simulink model "BoatSim"  (R2018a)
settings: Solver=ode45  StartTime=0.0  StopTime=50  RelTol=1e-3  EnableMultiTasking=on
values from neighbouring files (symbols this model uses):
  Dr = 30000    [BoatSim_config.m]
  Du = 1000    [BoatSim_config.m]
  Dv = 10000    [BoatSim_config.m]
  IoM = ( 1 / 5 ) * Mass * ( ( Length / 2 )^2 + ( Width / 2 )^2 )    (= 4143.75)    [BoatSim_config.m]
  Mass = 1500    [BoatSim_config.m]
  rg = [ 0;0; ]    [BoatSim_config.m]
undefined symbols (not defined in the file or in its folder): OM, sigbuilder_block
libraries: simulink x1
settings Model: Creator=hamada  LastModifiedBy=ryodo
settings DataIOCC: LimitDataPoints=on  SaveFormat=Array
settings OptimizationCC: LifeSpan=inf
settings DebuggingCC: SFUnexpectedBacktrackingDiag=warning  SFNoUnconditionalDefaultTransitionDiag=warning  SFExecutionAtInitializationDiag=none
settings HardwareCC: ProdBitPerPointer=32  ProdBitPerSizeT=32  ProdBitPerPtrDiffT=32  ProdLargestAtomicFloat=None  ProdIntDivRoundTo=Undefined  ProdEndianess=Unspecified  ProdWordSize=32  ProdHWDeviceType=32-bit Generic
settings ModelReferenceCC: PropagateSignalLabelsOutOfModel=off
settings CodeAppCC: StateflowObjectComments=on
settings GRTTargetCC: TargetLangStandard=C89/C90 (ANSI)  GeneratePreprocessorConditionals=Disable all
settings ConfigComp: CovMetricSettings=dw  CovHtmlReporting=on  CovSaveCumulativeToWorkspaceVar=on  CovSaveSingleToWorkspaceVar=on  CovExternalEMLEnable=off

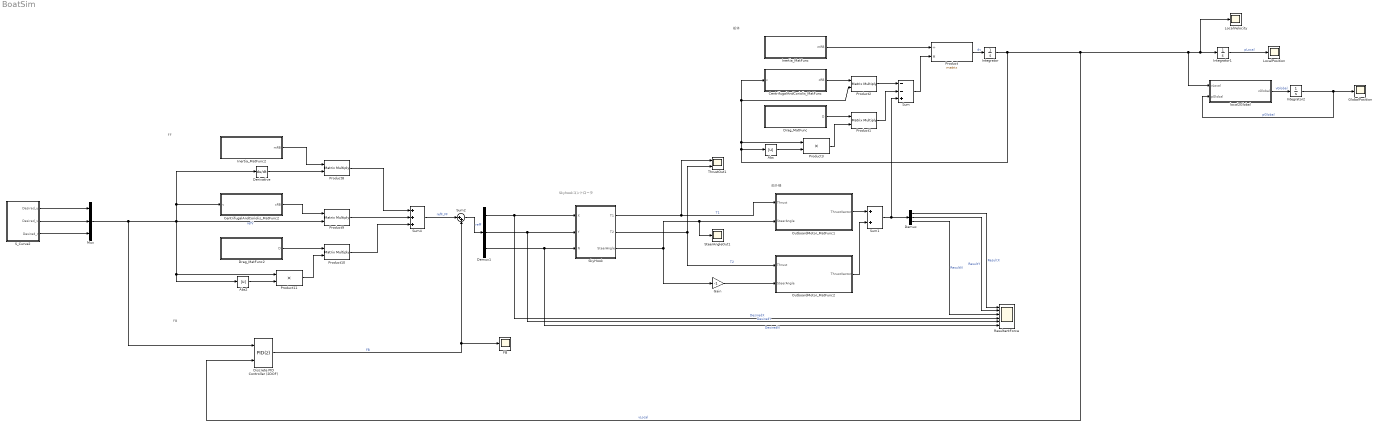
== system BoatSim ==
  note: 船外機
  note: 船体
  note: Skyhookコントローラ
  note: FF
  note: FB
  Abs : Abs
  Abs2 : Abs
  CentrifugalAndCoriolis_MatFunc : MATLAB Function  TreatAsAtomicUnit=on
  CentrifugalAndCoriolis_MatFunc2 : MATLAB Function  TreatAsAtomicUnit=on
  Demux : Demux  Outputs=3
  Demux1 : Demux  Outputs=3
  Derivative : Derivative
  Discrete PID Controller (2DOF) : simulink/Continuous/PID Controller (2DOF)  Controller=PID  TimeDomain=Discrete-time  SampleTime=-1  IntegratorMethod=Forward Euler  FilterMethod=Forward Euler  Form=Parallel  UseFilter=on  ControllerParametersSource=internal  P=1000  I=0  D=0  N=100  b=1  c=1  InitialConditionSource=internal  InitialConditionForIntegrator=0  InitialConditionForFilter=0  ExternalReset=none  ZeroCross=off  LimitOutput=off  UpperSaturationLimit=inf  LowerSaturationLimit=-inf  LinearizeAsGain=off  AntiWindupMode=none  Kb=1  TrackingMode=off  Kt=1  PParamMin=[]  PParamMax=[]  IParamMin=[]  IParamMax=[]  DParamMin=[]  DParamMax=[]  NParamMin=[]  NParamMax=[]  bParamMin=[]  bParamMax=[]  cParamMin=[]  cParamMax=[]  KbParamMin=[]  KbParamMax=[]  KtParamMin=[]  KtParamMax=[]  POutMin=[]  POutMax=[]  IOutMin=[]  IOutMax=[]  DOutMin=[]  DOutMax=[]  NOutMin=[]  NOutMax=[]  bOutMin=[]  bOutMax=[]  cOutMin=[]  cOutMax=[]  KbOutMin=[]  KbOutMax=[]  KtOutMin=[]  KtOutMax=[]  IntegratorOutMin=[]  IntegratorOutMax=[]  FilterOutMin=[]  FilterOutMax=[]  SumOutMin=[]  SumOutMax=[]  Sum1OutMin=[]  Sum1OutMax=[]  Sum2OutMin=[]  Sum2OutMax=[]  Sum3OutMin=[]  Sum3OutMax=[]  SumI1OutMin=[]  SumI1OutMax=[]  SumI2OutMin=[]  SumI2OutMax=[]  SumI3OutMin=[]  SumI3OutMax=[]  SumDOutMin=[]  SumDOutMax=[]  SaturationOutMin=[]  SaturationOutMax=[]  IntegratorContinuousStateAttributes=''  IntegratorStateMustResolveToSignalObject=off  IntegratorRTWStateStorageClass=Auto  FilterContinuousStateAttributes=''  FilterStateMustResolveToSignalObject=off  FilterRTWStateStorageClass=Auto  DifferentiatorICPrevScaledInput=0  DifferentiatorOutMin=[]  DifferentiatorOutMax=[]  FilterDiffOutCoefMin=[]  FilterDiffOutCoefMax=[]  SumDenOutMin=[]  SumDenOutMax=[]  SumNumOutMin=[]  SumNumOutMax=[]  ReciprocalOutMin=[]  ReciprocalOutMax=[]  DivideOutMin=[]  DivideOutMax=[]  TunerSelectOption=Transfer Function Based (PID Tuner App)
  Drag_MatFunc : MATLAB Function  TreatAsAtomicUnit=on  SystemSampleTime=0
      settings: MinAlgLoopOccurrences=on
  Drag_MatFunc2 : MATLAB Function  TreatAsAtomicUnit=on
  FB : Scope
  Gain : Gain  Gain=-1
  GlobalPosition : Scope
  Inertia_MatFunc : MATLAB Function  TreatAsAtomicUnit=on  SystemSampleTime=0
  Inertia_MatFunc2 : MATLAB Function  TreatAsAtomicUnit=on
  Integrator : Integrator
  Integrator1 : Integrator
  Integrator2 : Integrator
  LocalPosition : Scope
  "LocalVelocity " : Scope
  Mux : Mux  Inputs=3
  OutboardMotor_MatFunc1 : MATLAB Function  TreatAsAtomicUnit=on
  OutboardMotor_MatFunc2 : MATLAB Function  TreatAsAtomicUnit=on
  Product : Product  Inputs=/*  Multiplication=Matrix(*)
  Product{1..2,8..10} (5 alike) : Product  Multiplication=Matrix(*)
  Product11 : Product
  Product3 : Product
  ResultantForce : Scope  NumInputPorts=6
  S_Curve2 : Subsystem  Tag=STV Subsys  LoadFcn=sigbuilder_block('load',[244.8 146.274 948.126 560.842 ]);  StartFcn=sigbuilder_block('start');  StopFcn=sigbuilder_block('stop');  ClipboardFcn=sigbuilder_block('clipboard');  mask(Sigbuilder block){tuvar=[0:10]}
      mask help: Simulink:masks:SigbuilderBlock_MD
      mask init:
      | if ~strcmp(get_param(bdroot(gcbh),'SimulationStatus'),'stopped') tuvar = sigbuilder_block('maskInit'); end
      settings: CopyFcn=sigbuilder_block('copy');  DeleteFcn=sigbuilder_block('delete');  ModelCloseFcn=sigbuilder_block('modelClose');  PreSaveFcn=sigbuilder_block('preSave');  PauseFcn=sigbuilder_block('pause');  ContinueFcn=sigbuilder_block('continue');  NameChangeFcn=sigbuilder_block('namechange');  OpenFcn=sigbuilder_block('open',[674 298 550 400 ]);  CloseFcn=sigbuilder_block('close');
      mask Display: plot(0, 0, 100, 100,[2, 2, 32, 32, 2], [68, 8, 8, 68, 68],[32, 2], [38, 38], [32, 19, 2],[53, 60, 44], [32, 17, 17, 2],[16, 16, 31, 31]);txt = getActiveGroup(gcbh);text(2, 100, txt,'verticalAlignment', 'top');
  "SkyHook " : MATLAB Function  TreatAsAtomicUnit=on
  SteerAngleOut1 : Scope
  Sum : Sum  Inputs=--+
  Sum1 : Sum
  Sum2 : Sum  Inputs=|++
  Sum4 : Sum  Inputs=+++
  ThrustOut1 : Scope  NumInputPorts=2
  local2Global : MATLAB Function  TreatAsAtomicUnit=on
  wires:
  Inertia_MatFunc/1(mRB) -> Product/1
  Product/1 -> Integrator/1  "dv"
  Integrator/1 -> Discrete PID Controller (2DOF)/2, local2Global/1(vLocal), "LocalVelocity "/1, Integrator1/1, Abs/1, Product3/1, CentrifugalAndCoriolis_MatFunc/1(v), Product2/2  "vLocal"
  Integrator1/1 -> LocalPosition/1  "pLocal"
  CentrifugalAndCoriolis_MatFunc/1(cRB) -> Product2/1
  Product2/1 -> Sum/1
  Drag_MatFunc/1(D) -> Product1/1
  Sum/1 -> Product/2
  local2Global/1(vGlobal) -> Integrator2/1  "vGlobal"
  Integrator2/1 -> local2Global/2(pGlobal), GlobalPosition/1  "pGlobal"
  Sum1/1 -> Demux/1, Sum/3
  OutboardMotor_MatFunc1/1(ThrustVector) -> Sum1/1
  OutboardMotor_MatFunc2/1(ThrustVector) -> Sum1/2
  Demux/1 -> ResultantForce/1  "ResultX"
  Demux/2 -> ResultantForce/2  "ResultY"
  Demux/3 -> ResultantForce/3  "ResultN"
  Product1/1 -> Sum/2
  Product3/1 -> Product1/2
  Abs/1 -> Product3/2
  S_Curve2/1(Desired_u) -> Mux/1
  S_Curve2/2(Desired_v) -> Mux/2
  S_Curve2/3(Desired_r) -> Mux/3
  Inertia_MatFunc2/1(mRB) -> Product8/1
  Derivative/1 -> Product8/2
  CentrifugalAndCoriolis_MatFunc2/1(cRB) -> Product9/1
  Abs2/1 -> Product11/2
  Mux/1 -> Discrete PID Controller (2DOF)/1, Product11/1, Abs2/1, Derivative/1, CentrifugalAndCoriolis_MatFunc2/1(v), Product9/2  "refV"
  Product11/1 -> Product10/2
  Drag_MatFunc2/1(D) -> Product10/1
  Product8/1 -> Sum4/1
  Product9/1 -> Sum4/2
  Product10/1 -> Sum4/3
  Demux1/1 -> ResultantForce/4, "SkyHook "/1(X)  "DesiredX"
  Demux1/3 -> ResultantForce/6, "SkyHook "/3(N)  "DesiredN"
  Sum4/1 -> Sum2/1  "refF_FF"
  Demux1/2 -> "SkyHook "/2(Y), ResultantForce/5  "DesiredY"
  Sum2/1 -> Demux1/1  "refF"
  Discrete PID Controller (2DOF)/1 -> FB/1, Sum2/2  "FB"
  "SkyHook "/3(SteerAngle) -> SteerAngleOut1/1, OutboardMotor_MatFunc1/2(SteerAngle), Gain/1
  Gain/1 -> OutboardMotor_MatFunc2/2(SteerAngle)
  "SkyHook "/1(T1) -> ThrustOut1/1, OutboardMotor_MatFunc1/1(Thrust)  "T1"
  "SkyHook "/2(T2) -> ThrustOut1/2, OutboardMotor_MatFunc2/1(Thrust)  "T2"

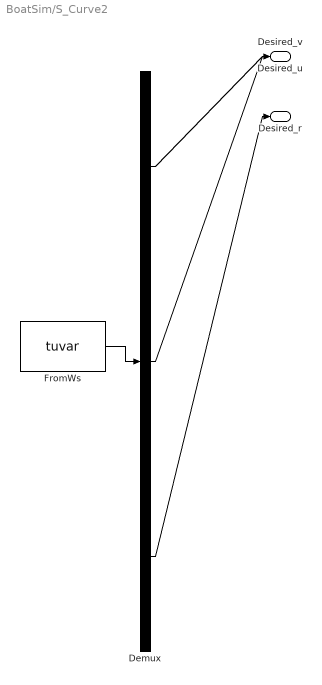
== system BoatSim/S_Curve2 ==
  Demux : Demux  Tag=STV Demux  Outputs=3
  FromWs : FromWorkspace  Tag=STV FromWs  VariableName=tuvar  SampleTime=0
      SigBuilderData=|
      | common.afterFinalStr = 'Extrapolate'
      | common.sampleTime = 0
      | dataSet(1).timeRange = [0 50]
      | dataSet(1).name = 'Group 2'
      | dataSet(2).timeRange = [0 50]
      | dataSet(2).name = 'Group 1'
      | dataSet(3).timeRange = [0 50]
      | dataSet(3).name = 'Group 3'
      | sbobj.Groups(1).Name = 'Group 2'
      | sbobj.Groups(1).Signals(1).Name = 'Desired_u'
      | sbobj.Groups(1).Signals(1).XData = [0 5 10 15 50]
      | sbobj.Groups(1).Signals(1).YData = [0 1 1 0 0]
      | sbobj.Groups(1).Signals(2).Name = 'Desired_v'
      | sbobj.Groups(1).Signals(2).XData = [0 20 25 30 35 50]
      | sbobj.Groups(1).Signals(2).YData = [0 0 0.1 0.1 0 0]
      | sbobj.Groups(1).Signals(3).Name = 'Desired_r'
      | sbobj.Groups(1).Signals(3).XData = [0 28 30 50]
      | sbobj.Groups(1).Signals(3).YData = [0 0.48 -0.215 0]
      | sbobj.Groups(1).TimeRange = [0 50]
      | sbobj.Groups(2).Name = 'Group 1'
      | sbobj.Groups(2).Signals(1).Name = 'Desired_u'
      | sbobj.Groups(2).Signals(1).XData = [0 1.05263157895 2.10526315789 3.15789473684 4.21052631579 5.26315789474 6.31578947368 7.36842105263 8.42105263158 9.47368421053 10.5263157895 11.5789473684 12.6315789474 13.6842105263 14.7368421053 15.7894736842 16.8421052632 17.8947368421 18.9473684211 20 21.0526315789 22.1052631579 23.1578947368 24.2105263158 25.2631578947 26.3157894737 27.3684210526 28.4210526316 29.4736842105 30.5263157895 31.5789473684 32.6315789474 33.6842105263 34.7368421053 35.7894736842 36.8421052632 37.8947368421 38.9473684211 40 41.0526315789 42.1052631579 43.1578947368 44.2105263158 45.2631578947 46.3157894737 47.3684210526 48.4210526316 49.4736842105 50]
      | sbobj.Groups(2).Signals(1).YData = [0 0.162349734602 0.307106356345 0.418583239131 0.48470013297 0.498292246503 0.457886663328 0.367861955337 0.237973696519 0.0822972951404 -0.0822972951404 -0.237973696519 -0.367861955337 -0.457886663328 -0.498292246503 -0.48470013297 -0.418583239131 -0.307106356345 -0.162349734602 0 0.162349734602 0.307106356345 0.418583239131 0.48470013297 0.498292246503 0.457886663328 0.367861955337 0.237973696519 0.0822972951404 -0.0822972951404 -0.237973696519 -0.367861955337 -0.457886663328 -0.498292246503 -0.48470013297 -0.418583239131 -0.307106356345 -0.162349734602 0 0.162349734602 0.307106356345 0.418583239131 0.48470013297 0.498292246503 0.457886663328 0.367861955337 0.237973696519 0.0822972951404 -5.82016719913e-16]
      | sbobj.Groups(2).Signals(2).Name = 'Desired_v'
      | sbobj.Groups(2).Signals(2).XData = [0 2.5641025641 5.12820512821 7.69230769231 10.2564102564 12.8205128205 15.3846153846 17.9487179487 20.5128205128 23.0769230769 25.641025641 28.2051282051 30.7692307692 33.3333333333 35.8974358974 38.4615384615 41.0256410256 43.5897435897 46.1538461538 48.7179487179 50]
      | sbobj.Groups(2).Signals(2).YData = [0 0.0160411280858 0.0316667993801 0.0464723172044 0.0600742264238 0.0721202447344 0.0822983865894 0.090345043461 0.0960518111631 0.0992708874098 0.0999188998172 0.0979790652042 0.0935016242685 0.0866025403784 0.0774604961828 0.0663122658241 0.0534465826128 0.039196660986 0.0239315664288 0.00804665687167 1.22464679915e-17]
      | sbobj.Groups(2).Signals(3).Name = 'Desired_r'
      | sbobj.Groups(2).Signals(3).XData = [0 1.28205128205 2.5641025641 3.84615384615 5.12820512821 6.41025641026 7.69230769231 8.97435897436 10.2564102564 11.5384615385 12.8205128205 14.1025641026 15.3846153846 16.6666666667 17.9487179487 19.2307692308 20.5128205128 21.7948717949 23.0769230769 24.358974359 25.641025641 26.9230769231 28.2051282051 29.4871794872 30.7692307692 32.0512820513 33.3333333333 34.6153846154 35.8974358974 37.1794871795 38.4615384615 39.7435897436 41.0256410256 42.3076923077 43.5897435897 44.8717948718 46.1538461538 47.4358974359 48.7179487179 50]
      | sbobj.Groups(2).Signals(3).YData = [0 0.0160411280858 0.0316667993801 0.0464723172044 0.0600742264238 0.0721202447344 0.0822983865894 0.090345043461 0.0960518111631 0.0992708874098 0.0999188998172 0.0979790652042 0.0935016242685 0.0866025403784 0.0774604961828 0.0663122658241 0.0534465826128 0.039196660986 0.0239315664288 0.00804665687167 -0.00804665687167 -0.0239315664288 -0.039196660986 -0.0534465826128 -0.0663122658241 -0.0774604961828 -0.0866025403784 -0.0935016242685 -0.0979790652042 -0.0999188998172 -0.0992708874098 -0.0960518111631 -0.090345043461 -0.0822983865894 -0.0721202447344 -0.0600742264238 -0.0464723172044 -0.0316667993801 -0.0160411280858 0]
      | sbobj.Groups(2).TimeRange = [0 50]
      | sbobj.Groups(3).Name = 'Group 3'
      | sbobj.Groups(3).Signals(1).Name = 'Desired_u'
      | sbobj.Groups(3).Signals(1).XData = [0 5.26315789474 10.5263157895 15.7894736842 21.0526315789 26.3157894737 31.5789473684 36.8421052632 42.1052631579 47.3684210526 50]
      | sbobj.Groups(3).Signals(1).YData = [0 0.324699469205 0.61421271269 0.837166478263 0.969400265939 0.996584493007 0.915773326655 0.735723910673 0.475947393037 0.164594590281 1.22464679915e-16]
      | sbobj.Groups(3).Signals(2).Name = 'Desired_v'
      | sbobj.Groups(3).Signals(2).XData = [0 0.526315789474 1.05263157895 1.57894736842 2.10526315789 2.63157894737 3.15789473684 3.68421052632 4.21052631579 4.73684210526 5.26315789474 5.78947368421 6.31578947368 6.84210526316 7.36842105263 7.89473684211 8.42105263158 8.94736842105 9.47368421053 10 10.5263157895 11.0526315789 11.5789473684 12.1052631579 12.6315789474 13.1578947368 13.6842105263 14.2105263158 14.7368421053 15.2631578947 15.7894736842 16.3157894737 16.8421052632 17.3684210526 17.8947368421 18.4210526316 18.9473684211 19.4736842105 20 20.5263157895 21.0526315789 21.5789473684 22.1052631579 22.6315789474 23.1578947368 23.6842105263 24.2105263158 24.7368421053 25.2631578947 25.7894736842 26.3157894737 26.8421052632 27.3684210526 27.8947368421 28.4210526316 28.9473684211 29.4736842105 30 30.5263157895 31.0526315789 31.5789473684 32.1052631579 32.6315789474 33.1578947368 33.6842105263 34.2105263158 34.7368421053 35.2631578947 35.7894736842 36.3157894737 36.8421052632 37.3684210526 37.8947368421 38.4210526316 38.9473684211 39.4736842105 40 40.5263157895 41.0526315789 41.5789473684 42.1052631579 42.6315789474 43.1578947368 43.6842105263 44.2105263158 44.7368421053 45.2631578947 45.7894736842 46.3157894737 46.8421052632 47.3684210526 47.8947368421 48.4210526316 48.9473684211 49.4736842105 50]
      | sbobj.Groups(3).Signals(2).YData = [0 0.0162349734602 0.0307106356345 0.0418583239131 0.048470013297 0.0498292246503 0.0457886663328 0.0367861955337 0.0237973696519 0.00822972951404 -0.00822972951404 -0.0237973696519 -0.0367861955337 -0.0457886663328 -0.0498292246503 -0.048470013297 -0.0418583239131 -0.0307106356345 -0.0162349734602 0 0.0162349734602 0.0307106356345 0.0418583239131 0.048470013297 0.0498292246503 0.0457886663328 0.0367861955337 0.0237973696519 0.00822972951404 -0.00822972951404 -0.0237973696519 -0.0367861955337 -0.0457886663328 -0.0498292246503 -0.048470013297 -0.0418583239131 -0.0307106356345 -0.0162349734602 0 0.0162349734602 0.0307106356345 0.0418583239131 0.048470013297 0.0498292246503 0.0457886663328 0.0367861955337 0.0237973696519 0.00822972951404 -0.00822972951404 -0.0237973696519 -0.0367861955337 -0.0457886663328 -0.0498292246503 -0.048470013297 -0.0418583239131 -0.0307106356345 -0.0162349734602 0 0.0162349734602 0.0307106356345 0.0418583239131 0.048470013297 0.0498292246503 0.0457886663328 0.0367861955337 0.0237973696519 0.00822972951404 -0.00822972951404 -0.0237973696519 -0.0367861955337 -0.0457886663328 -0.0498292246503 -0.048470013297 -0.0418583239131 -0.0307106356345 -0.0162349734602 0 0.0162349734602 0.0307106356345 0.0418583239131 0.048470013297 0.0498292246503 0.0457886663328 0.0367861955337 0.0237973696519 0.00822972951404 -0.00822972951404 -0.0237973696519 -0.0367861955337 -0.0457886663328 -0.0498292246503 -0.048470013297 -0.0418583239131 -0.0307106356345 -0.0162349734602 0]
      | sbobj.Groups(3).Signals(3).Name = 'Desired_r'
      | sbobj.Groups(3).Signals(3).XData = [0 28 30 50]
      | sbobj.Groups(3).Signals(3).YData = [0 0.08 -0.14 0]
      | sbobj.Groups(3).TimeRange = [0 50]
  Desired_u : Outport  Tag=STV Outport
  Desired_v : Outport  Tag=STV Outport  Port=2
  Desired_r : Outport  Tag=STV Outport  Port=3
  wires:
  FromWs/1 -> Demux/1
  Demux/1 -> Desired_u/1
  Demux/2 -> Desired_v/1
  Demux/3 -> Desired_r/1

== matlab function BoatSim/CentrifugalAndCoriolis_MatFunc ==
  data: v input size=3; Mass parameter size=1; rg parameter size=2; cRB output size=3,3
function cRB = CentrifugalAndCoriolis_MatFunc( v, Mass, rg )
    cRB = CentrifugalAndCoriolis( Mass, rg, v );
end

== matlab function BoatSim/Inertia_MatFunc ==
  data: Mass parameter size=1; mRB output size=3,3; IoM parameter size=1; rg parameter size=2
function mRB = Inertia_MatFunc( Mass, IoM, rg )
    mRB = Inertia( Mass, IoM, rg );
end

== matlab function BoatSim/Drag_MatFunc ==
  data: Du parameter size=1; Dv parameter size=1; D output size=3,3; Dr parameter size=1
function D = Drag_MatFunc( Du, Dv, Dr )
    D = Drag( Du, Dv, Dr );
end

== matlab function BoatSim/local2Global ==
  data: vLocal input size=3; vGlobal output size=3; pGlobal input size=3
function vGlobal = local2global_MatFunc( vLocal, pGlobal )
    vGlobal = local2global( vLocal, pGlobal );
end

== matlab function BoatSim/OutboardMotor_MatFunc1 ==
  data: Thrust input size=2; ThrustVector output size=3; SteerAngle input size=1; rg parameter size=2; OM parameter
function ThrustVector = OutboardMotor_MatFunc( Thrust, SteerAngle, rg, OM )
    ThrustVector = OutboardMotor( Thrust, SteerAngle, rg, OM(1).rb2om );
end

== matlab function BoatSim/OutboardMotor_MatFunc2 ==
  data: Thrust input size=2; ThrustVector output size=3; SteerAngle input size=1; rg parameter size=2; OM parameter
function ThrustVector = OutboardMotor_MatFunc( Thrust, SteerAngle, rg, OM )
    ThrustVector = OutboardMotor( Thrust, SteerAngle, rg, OM(2).rb2om );
end

== matlab function BoatSim/SkyHook  ==
  data: X input double size=1; T1 output double size=2; Y input double size=1; N input double size=1; T2 output double size=2; SteerAngle output double size=1
function [ T1, T2, SteerAngle ]  = SkyHook_MatFunc(X, Y, N)
    rx = 3;%OM(1).rb2om(1);
    ry = 0.5;%OM(1).rb2om(2);
    if Y == 0 % sin=0
        SteerAngle = 0;
        T1 = [(X + N/ry) / 2; 0;];
        T2 = [(X - N/ry) / 2; 0;];
    elseif Y*rx+N == 0 % cos=0
        SteerAngle = 0; % pi/2;
        T1 = [0;0;];
        T2 = [0;0;];
    else
        SteerAngle = atan(ry*Y / (rx*Y+N)); % -pi/2 < SteerAngle < pi/2
        Tplus = X / cos(SteerAngle);
        Tminus = Y / sin(SteerAngle);
        T1 = [(Tplus + Tminus) / 2; 0;];
        T2 = [(Tplus - Tminus) / 2; 0;];
    end
    
end

== matlab function BoatSim/Inertia_MatFunc2 ==
  data: Mass parameter size=1; mRB output size=3,3; IoM parameter size=1; rg parameter size=2
function mRB = Inertia_MatFunc( Mass, IoM, rg )
    mRB = Inertia( Mass, IoM, rg );
end

== matlab function BoatSim/CentrifugalAndCoriolis_MatFunc2 ==
  data: v input size=3; Mass parameter size=1; rg parameter size=2; cRB output size=3,3
function cRB = CentrifugalAndCoriolis_MatFunc( v, Mass, rg )
    cRB = CentrifugalAndCoriolis( Mass, rg, v );
end

== matlab function BoatSim/Drag_MatFunc2 ==
  data: Du parameter size=1; Dv parameter size=1; D output size=3,3; Dr parameter size=1
function D = Drag_MatFunc( Du, Dv, Dr )
    D = Drag( Du, Dv, Dr );
end
